simulink model "USV_ASMC"  (R2019b)
settings: Solver=ode1  StartTime=0.0  StopTime=70  FixedStep=0.01  RelTol=1e-3
undefined symbols (not defined in the file): sigbuilder_block
libraries: sharedutil x6, simulink_extras x2, simulink x2, aerolibutil x1
settings Model: Creator=Alex Glz  LastModifiedBy=alex
settings SolverCC: ZeroCrossAlgorithm=Adaptive
settings DataIOCC: ReturnWorkspaceOutputs=off
settings DebuggingCC: IgnoredZcDiagnostic=none  PregeneratedLibrarySubsystemCodeDiagnostic=none  ArithmeticOperatorsInVariantConditions=warning
settings SFSimCC: SimUseLocalCustomCode=off  CustomCodeUndefinedFunction=UseInterfaceOnly
settings RTWCC: RTWUseLocalCustomCode=off

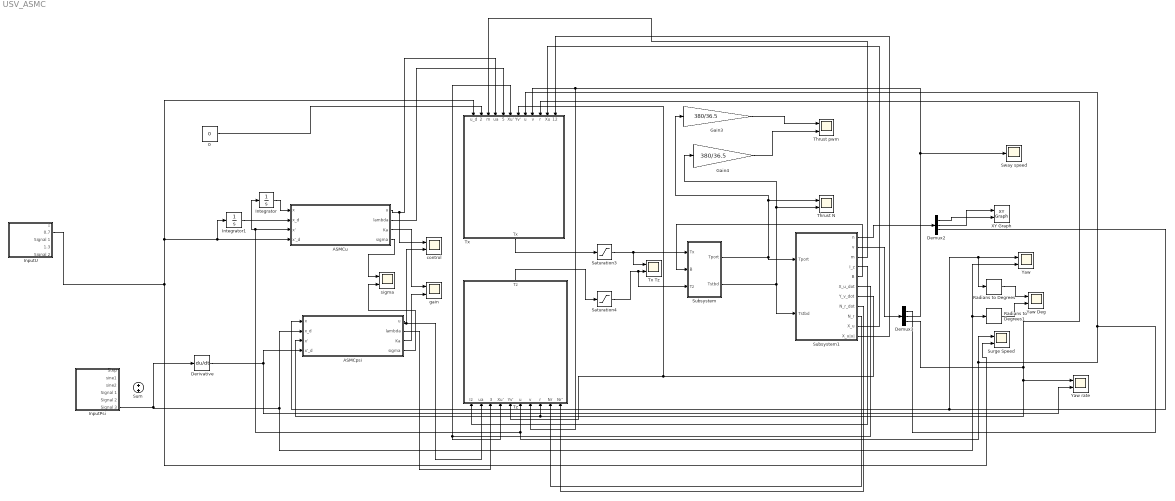
== system USV_ASMC ==
  0 : Constant  Value=0  SampleTime=Inf
  ASMCpsi : Subsystem
  ASMCu : Subsystem
  Demux2 : Demux  Outputs=3
  Demux3 : Demux  Outputs=3
  Derivative : Derivative
  Gain3 : Gain  Gain=380/36.5
  Gain4 : Gain  Gain=380/36.5
  InputPsi : Subsystem  Tag=STV Subsys  LoadFcn=sigbuilder_block('load');  StartFcn=sigbuilder_block('start');  StopFcn=sigbuilder_block('stop');  ClipboardFcn=sigbuilder_block('clipboard');  mask(Sigbuilder block){tuvar=[0:10]}
      mask help: Simulink:masks:SigbuilderBlock_MD
      mask init:
      | if ~strcmp(get_param(bdroot(gcbh),'SimulationStatus'),'stopped') tuvar = sigbuilder_block('maskInit'); end
      settings: CopyFcn=sigbuilder_block('copy');  DeleteFcn=sigbuilder_block('delete');  ModelCloseFcn=sigbuilder_block('modelClose');  PreSaveFcn=sigbuilder_block('preSave');  PauseFcn=sigbuilder_block('pause');  ContinueFcn=sigbuilder_block('continue');  NameChangeFcn=sigbuilder_block('namechange');  OpenFcn=sigbuilder_block('open',[327.411 0 679.074 714.695 ]);  CloseFcn=sigbuilder_block('close');
      mask Display: plot(0, 0, 100, 100,[2, 2, 32, 32, 2], [68, 8, 8, 68, 68],[32, 2], [38, 38], [32, 19, 2],[53, 60, 44], [32, 17, 17, 2],[16, 16, 31, 31]);txt = getActiveGroup(gcbh);text(2, 100, txt,'verticalAlignment', 'top');
  InputU : Subsystem  Tag=STV Subsys  LoadFcn=sigbuilder_block('load');  StartFcn=sigbuilder_block('start');  StopFcn=sigbuilder_block('stop');  ClipboardFcn=sigbuilder_block('clipboard');  mask(Sigbuilder block){tuvar=[0:10]}
      mask help: Simulink:masks:SigbuilderBlock_MD
      mask init:
      | if ~strcmp(get_param(bdroot(gcbh),'SimulationStatus'),'stopped') tuvar = sigbuilder_block('maskInit'); end
      settings: CopyFcn=sigbuilder_block('copy');  DeleteFcn=sigbuilder_block('delete');  ModelCloseFcn=sigbuilder_block('modelClose');  PreSaveFcn=sigbuilder_block('preSave');  PauseFcn=sigbuilder_block('pause');  ContinueFcn=sigbuilder_block('continue');  NameChangeFcn=sigbuilder_block('namechange');  OpenFcn=sigbuilder_block('open',[122.021 0 701.053 737.432 ]);  CloseFcn=sigbuilder_block('close');
      mask Display: plot(0, 0, 100, 100,[2, 2, 32, 32, 2], [68, 8, 8, 68, 68],[32, 2], [38, 38], [32, 19, 2],[53, 60, 44], [32, 17, 17, 2],[16, 16, 31, 31]);txt = getActiveGroup(gcbh);text(2, 100, txt,'verticalAlignment', 'top');
  Integrator : Integrator
  Integrator1 : Integrator
  Radians to Degrees : simulink_extras/Transformations/Radians to Degrees
  Radians to Degrees1 : simulink_extras/Transformations/Radians to Degrees
  Saturation3 : Saturate  UpperLimit=64.97  LowerLimit=-64.97
  Saturation4 : Saturate  UpperLimit=13.31  LowerLimit=-13.31
  Subsystem : Subsystem
  Subsystem1 : Subsystem
  Sum : Sum
  Surge Speed : Scope  NumInputPorts=2
  Sway speed : Scope
  Thrust N : Scope  NumInputPorts=2
  Thrust pwm : Scope  NumInputPorts=2
  Tx : Subsystem
  Tx Tz : Scope  NumInputPorts=2
  Tz : Subsystem
  XY Graph : simulink/Sinks/XY Graph  xmin=-20  xmax=20  ymin=-5  ymax=100  st=-1
  Yaw : Scope  NumInputPorts=2
  Yaw Deg : Scope  NumInputPorts=2
  Yaw rate : Scope  NumInputPorts=2
  control : Scope  NumInputPorts=2
  gain : Scope  NumInputPorts=2
  sigma : Scope  NumInputPorts=2
  wires:
  Subsystem1/1(n) -> Demux2/1
  Subsystem1/2(v) -> Demux3/1
  Gain4/1 -> Thrust pwm/2
  Gain3/1 -> Thrust pwm/1
  Derivative/1 -> ASMCpsi/4(x'_d), Yaw rate/2
  InputU/2(0.7) -> Surge Speed/2, Tx/1(u_d), ASMCu/4(x'_d), Integrator1/1
  Subsystem/2(Tstbd) -> Subsystem1/2(Tstbd), Gain4/1, Thrust N/2
  Subsystem/1(Tport) -> Subsystem1/1(Tport), Thrust N/1, Gain3/1
  Subsystem1/5(B) -> Subsystem/2(B)
  Subsystem1/3(m) -> Tx/3(m)
  ASMCu/1(u) -> control/1, Tx/4(ua)
  ASMCu/2(lambda) -> Tx/5(lambda)
  Subsystem1/6(X_u_dot) -> Tz/4(Xu'), Tx/6(Xu')
  Subsystem1/7(Y_v_dot) -> Tz/5(Yv'), Tx/7(Yv')
  Demux3/1 -> Surge Speed/1, Integrator/1, ASMCu/3(x'), Tz/6(u), Tx/8(u)
  Demux3/2 -> Sway speed/1, Tx/9(v), Tz/7(v)
  Demux3/3 -> Tz/8(r), ASMCpsi/3(x'), Yaw rate/1, Tx/10(r)
  Subsystem1/10(X_u) -> Tx/11(Xu)
  Subsystem1/11(X_u|u|) -> Tx/12(Xu|u|)
  Tx/1(Tx) -> Saturation3/1
  0/1 -> Tx/2(u'_d)
  Subsystem1/4(I_z) -> Tz/1(Iz)
  ASMCpsi/1(u) -> control/2, Tz/2(ua)
  ASMCpsi/2(lambda) -> Tz/3(lambda)
  Subsystem1/9(N_r) -> Tz/9(Nr)
  Subsystem1/8(N_r_dot) -> Tz/10(Nr')
  Tz/1(Tz) -> Saturation4/1
  Demux2/2 -> XY Graph/1
  Demux2/1 -> XY Graph/2
  Radians to Degrees/1 -> Yaw Deg/1
  Radians to Degrees1/1 -> Yaw Deg/2
  Demux2/3 -> Radians to Degrees/1, Yaw/1, ASMCpsi/1(x)
  ASMCu/3(Ka) -> gain/1
  ASMCpsi/3(Ka) -> gain/2
  ASMCu/4(sigma) -> sigma/1
  ASMCpsi/4(sigma) -> sigma/2
  Integrator1/1 -> ASMCu/2(x_d)
  Integrator/1 -> ASMCu/1(x)
  Saturation4/1 -> Subsystem/3(Tz), Tx Tz/2
  Saturation3/1 -> Subsystem/1(Tx), Tx Tz/1
  InputPsi/6(Signal 3) -> ASMCpsi/2(x_d), Yaw/2, Radians to Degrees1/1, Derivative/1

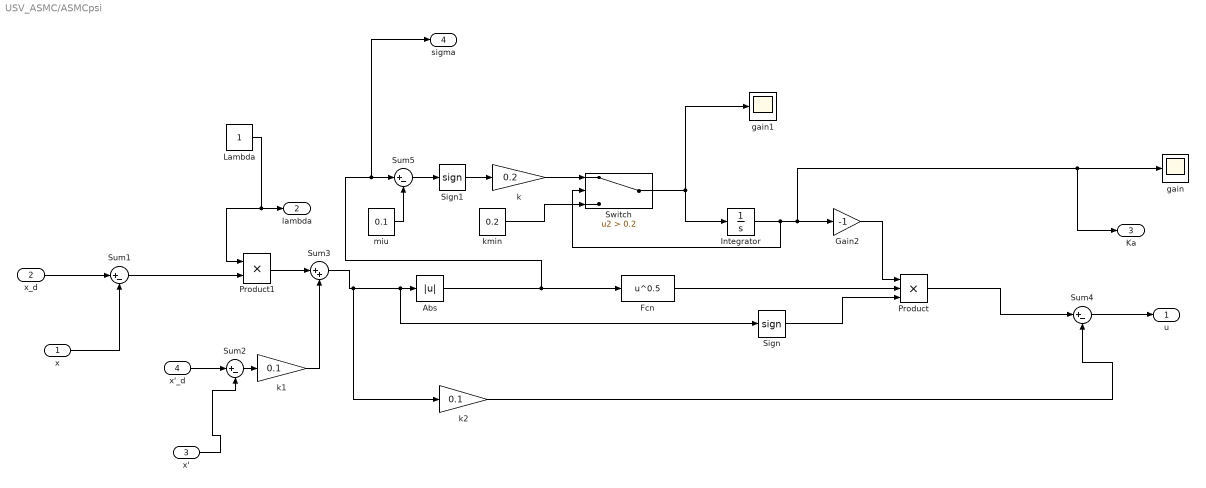
== system USV_ASMC/ASMCpsi ==
  x : Inport
  x_d : Inport  Port=2
  x' : Inport  Port=3
  x'_d : Inport  Port=4
  Abs : Abs
  Fcn : Fcn  Expr=u^0.5
  Gain2 : Gain  Gain=-1
  Integrator : Integrator
  Lambda : Constant
  Product : Product  Inputs=3
  Product1 : Product
  Sign : Signum
  Sign1 : Signum
  Sum{1..2,4..5} (4 alike) : Sum  Inputs=|+-
  Sum3 : Sum  Inputs=|++
  Switch : Switch  Criteria=u2 > Threshold  Threshold=0.2
  gain : Scope
  gain1 : Scope
  k : Gain  Gain=0.2
  k1 : Gain  Gain=0.1
  k2 : Gain  Gain=0.1
  kmin : Constant  Value=0.2
  miu : Constant  Value=0.1
  u : Outport  VectorParamsAs1DForOutWhenUnconnected=off
  lambda : Outport  Port=2  VectorParamsAs1DForOutWhenUnconnected=off
  Ka : Outport  Port=3  VectorParamsAs1DForOutWhenUnconnected=off
  sigma : Outport  Port=4  VectorParamsAs1DForOutWhenUnconnected=off
  wires:
  Product1/1 -> Sum3/1
  x'/1 -> Sum2/2
  x'_d/1 -> Sum2/1
  x_d/1 -> Sum1/1
  x/1 -> Sum1/2
  Sum4/1 -> u/1
  k2/1 -> Sum4/2
  Sum3/1 -> k2/1, Sign/1, Abs/1
  Product/1 -> Sum4/1
  Fcn/1 -> Product/2
  Sign/1 -> Product/3
  Gain2/1 -> Product/1
  Integrator/1 -> Switch/2, Ka/1, gain/1, Gain2/1
  miu/1 -> Sum5/2
  Sum5/1 -> Sign1/1
  Sign1/1 -> k/1
  k/1 -> Switch/1
  Switch/1 -> gain1/1, Integrator/1
  kmin/1 -> Switch/3
  Lambda/1 -> Product1/1, lambda/1
  Sum1/1 -> Product1/2
  Sum2/1 -> k1/1
  Abs/1 -> sigma/1, Sum5/1, Fcn/1
  k1/1 -> Sum3/2

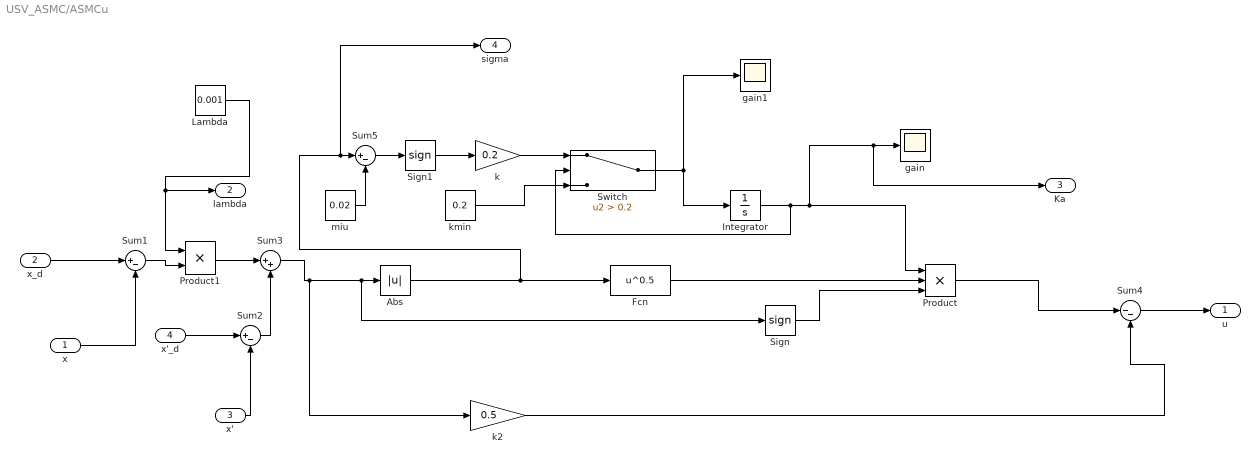
== system USV_ASMC/ASMCu ==
  x : Inport
  x_d : Inport  Port=2
  x' : Inport  Port=3
  x'_d : Inport  Port=4
  Abs : Abs
  Fcn : Fcn  Expr=u^0.5
  Integrator : Integrator
  Lambda : Constant  Value=0.001
  Product : Product  Inputs=3
  Product1 : Product
  Sign : Signum
  Sign1 : Signum
  Sum1 : Sum  Inputs=|+-
  Sum2 : Sum  Inputs=|+-
  Sum3 : Sum  Inputs=|++
  Sum4 : Sum  Inputs=|--
  Sum5 : Sum  Inputs=|+-
  Switch : Switch  Criteria=u2 > Threshold  Threshold=0.2
  gain : Scope
  gain1 : Scope
  k : Gain  Gain=0.2
  k2 : Gain  Gain=0.5
  kmin : Constant  Value=0.2
  miu : Constant  Value=0.02
  u : Outport  VectorParamsAs1DForOutWhenUnconnected=off
  lambda : Outport  Port=2  VectorParamsAs1DForOutWhenUnconnected=off
  Ka : Outport  Port=3  VectorParamsAs1DForOutWhenUnconnected=off
  sigma : Outport  Port=4  VectorParamsAs1DForOutWhenUnconnected=off
  wires:
  Product1/1 -> Sum3/1
  x'/1 -> Sum2/2
  x'_d/1 -> Sum2/1
  Sum2/1 -> Sum3/2
  x_d/1 -> Sum1/1
  x/1 -> Sum1/2
  Sum1/1 -> Product1/2
  Sum4/1 -> u/1
  k2/1 -> Sum4/2
  Sum3/1 -> k2/1, Sign/1, Abs/1
  Product/1 -> Sum4/1
  Fcn/1 -> Product/2
  Sign/1 -> Product/3
  Integrator/1 -> Switch/2, Product/1, Ka/1, gain/1
  miu/1 -> Sum5/2
  Sum5/1 -> Sign1/1
  Sign1/1 -> k/1
  k/1 -> Switch/1
  Switch/1 -> gain1/1, Integrator/1
  kmin/1 -> Switch/3
  Lambda/1 -> lambda/1, Product1/1
  Abs/1 -> sigma/1, Sum5/1, Fcn/1

== system USV_ASMC/InputPsi ==
  Demux : Demux  Tag=STV Demux  Outputs=6
  FromWs : FromWorkspace  Tag=STV FromWs  VariableName=tuvar  SampleTime=0
      SigBuilderData=|
      | common.afterFinalStr = 'Extrapolate'
      | common.sampleTime = 0
      | dataSet.timeRange = [0 90]
      | dataSet.name = 'Group 1'
      | sbobj.Groups.Name = 'Group 1'
      | sbobj.Groups.Signals(1).Name = 'Step'
      | sbobj.Groups.Signals(1).XData = [0 90]
      | sbobj.Groups.Signals(1).YData = [0.4 0.4]
      | sbobj.Groups.Signals(2).Name = 'sine1'
      | sbobj.Groups.Signals(2).XData = [0 2.94117647059 5.88235294118 8.82352941176 11.7647058824 14.7058823529 17.6470588235 20.5882352941 23.5294117647 26.4705882353 29.4117647059 32.3529411765 35.2941176471 38.2352941176 41.1764705882 44.1176470588 47.0588235294 50 90]
      | sbobj.Groups.Signals(2).YData = [0 0.144496666475 0.269478257459 0.358065316542 0.398293670518 0.384730257269 0.319206890912 0.210572865151 0.0734998071266 -0.0734998071266 -0.210572865151 -0.319206890912 -0.384730257269 -0.398293670518 -0.358065316542 -0.269478257459 -0.144496666475 0 0]
      | sbobj.Groups.Signals(3).Name = 'sine2'
      | sbobj.Groups.Signals(3).XData = [0 2.94117647059 5.88235294118 8.82352941176 11.7647058824 14.7058823529 17.6470588235 20.5882352941 23.5294117647 26.4705882353 29.4117647059 32.3529411765 35.2941176471 38.2352941176 41.1764705882 44.1176470588 45 50 90]
      | sbobj.Groups.Signals(3).YData = [0 0.0722483332374 0.134739128729 0.179032658271 0.199146835259 0.192365128635 0.159603445456 0.105286432575 0.0367499035633 -0.0367499035633 -0.105286432575 -0.159603445456 -0.192365128635 -0.199146835259 -0.179032658271 -0.134739128729 -0.117557050458 0 0]
      | sbobj.Groups.Signals(4).Name = 'Signal 1'
      | sbobj.Groups.Signals(4).XData = [0 30 30 50 60 60 90]
      | sbobj.Groups.Signals(4).YData = [3 3 2 2 2 1 1]
      | sbobj.Groups.Signals(5).Name = 'Signal 2'
      | sbobj.Groups.Signals(5).XData = [0 0.01 0.02 0.03 0.04 0.05 0.06 0.07 0.08 0.09 0.1 0.11 ... (9001 elements, 1x9001)]
      | sbobj.Groups.Signals(5).YData = [-0.0197341459996 0.0101006698948 0.00109159685548 0.00682613120581 -0.00894223767885 0.0161354484461 -0.00589998785907 0.00664245185836 -0.0112621395209 -0.00996625777906 -0.00906837882606 -0.00281492525369 ... (9001 elements, 1x9001)]
      | sbobj.Groups.Signals(6).Name = 'Signal 3'
      | sbobj.Groups.Signals(6).XData = [0 0.0625625625626 0.125125125125 0.187687687688 0.25025025025 0.312812812813 0.375375375375 0.437937937938 0.500500500501 0.563063063063 0.625625625626 0.688188188188 ... (1440 elements, 1x1440)]
      | sbobj.Groups.Signals(6).YData = [0 0.0157235832902 0.0314465445969 0.0471682619612 0.0628881134734 0.0786054772978 0.0943197316968 0.110030255056 0.125736425908 0.141437622959 0.157133225111 0.172822611487 ... (1440 elements, 1x1440)]
      | sbobj.Groups.TimeRange = [0 90]
  Step : Outport  Tag=STV Outport  VectorParamsAs1DForOutWhenUnconnected=off
  sine1 : Outport  Tag=STV Outport  Port=2  VectorParamsAs1DForOutWhenUnconnected=off
  sine2 : Outport  Tag=STV Outport  Port=3  VectorParamsAs1DForOutWhenUnconnected=off
  Signal 1 : Outport  Tag=STV Outport  Port=4  VectorParamsAs1DForOutWhenUnconnected=off
  Signal 2 : Outport  Tag=STV Outport  Port=5  VectorParamsAs1DForOutWhenUnconnected=off
  Signal 3 : Outport  Tag=STV Outport  Port=6
  wires:
  FromWs/1 -> Demux/1
  Demux/1 -> Step/1
  Demux/2 -> sine1/1
  Demux/3 -> sine2/1
  Demux/4 -> Signal 1/1
  Demux/5 -> Signal 2/1
  Demux/6 -> Signal 3/1

== system USV_ASMC/InputU ==
  Demux : Demux  Tag=STV Demux  Outputs=5
  FromWs : FromWorkspace  Tag=STV FromWs  VariableName=tuvar  SampleTime=0
      SigBuilderData=|
      | common.afterFinalStr = 'Extrapolate'
      | common.sampleTime = 0
      | dataSet.timeRange = [0 45]
      | dataSet.name = 'Group 1'
      | sbobj.Groups.Name = 'Group 1'
      | sbobj.Groups.Signals(1).Name = '1'
      | sbobj.Groups.Signals(1).XData = [0 45]
      | sbobj.Groups.Signals(1).YData = [1 1]
      | sbobj.Groups.Signals(2).Name = '0.7'
      | sbobj.Groups.Signals(2).XData = [0 45]
      | sbobj.Groups.Signals(2).YData = [0.7 0.7]
      | sbobj.Groups.Signals(3).Name = 'Signal 1'
      | sbobj.Groups.Signals(3).XData = [0 2.94117647059 5.88235294118 8.82352941176 11.7647058824 14.7058823529 17.6470588235 20.5882352941 23.5294117647 26.4705882353 29.4117647059 32.3529411765 35.2941176471 38.2352941176 41.1764705882 44.1176470588 45]
      | sbobj.Groups.Signals(3).YData = [0 0.680620833094 0.836847821823 0.947581645678 0.997867088148 0.980912821586 0.89900861364 0.763216081439 0.591874758908 0.408125241092 0.236783918561 0.10099138636 0.0190871784136 0 0 0 0]
      | sbobj.Groups.Signals(4).Name = '1.3'
      | sbobj.Groups.Signals(4).XData = [0 45]
      | sbobj.Groups.Signals(4).YData = [1.3 1.3]
      | sbobj.Groups.Signals(5).Name = 'Signal 2'
      | sbobj.Groups.Signals(5).XData = [0 2.94117647059 5.88235294118 8.82352941176 11.7647058824 14.7058823529 17.6470588235 20.5882352941 23.5294117647 26.4705882353 45]
      | sbobj.Groups.Signals(5).YData = [0 0.680620833094 0.836847821823 0.947581645678 0.997867088148 0.980912821586 0.89900861364 0.763216081439 0.591874758908 0.5 0.5]
      | sbobj.Groups.TimeRange = [0 45]
  1 : Outport  Tag=STV Outport  VectorParamsAs1DForOutWhenUnconnected=off
  0.7 : Outport  Tag=STV Outport  Port=2  VectorParamsAs1DForOutWhenUnconnected=off
  Signal 1 : Outport  Tag=STV Outport  Port=3  VectorParamsAs1DForOutWhenUnconnected=off
  1.3 : Outport  Tag=STV Outport  Port=4  VectorParamsAs1DForOutWhenUnconnected=off
  Signal 2 : Outport  Tag=STV Outport  Port=5  VectorParamsAs1DForOutWhenUnconnected=off
  wires:
  FromWs/1 -> Demux/1
  Demux/1 -> 1/1
  Demux/2 -> 0.7/1
  Demux/3 -> Signal 1/1
  Demux/4 -> 1.3/1
  Demux/5 -> Signal 2/1

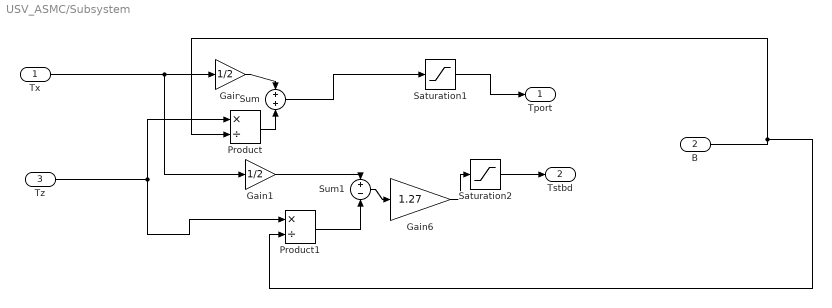
== system USV_ASMC/Subsystem ==
  Tx : Inport
  B : Inport  Port=2
  Tz : Inport  Port=3
  Gain : Gain  Gain=1/2
  Gain1 : Gain  Gain=1/2
  Gain6 : Gain  Gain=1.27
  Product : Product  Inputs=*/
  Product1 : Product  Inputs=*/
  Saturation1 : Saturate  UpperLimit=36.5  LowerLimit=-30
  Saturation2 : Saturate  UpperLimit=36.5  LowerLimit=-30
  Sum : Sum
  Sum1 : Sum  Inputs=+-
  Tport : Outport  VectorParamsAs1DForOutWhenUnconnected=off
  Tstbd : Outport  Port=2  VectorParamsAs1DForOutWhenUnconnected=off
  wires:
  Gain6/1 -> Saturation2/1
  Gain/1 -> Sum/1
  Sum/1 -> Saturation1/1
  B/1 -> Product/2, Product1/2
  Tz/1 -> Product1/1, Product/1
  Saturation1/1 -> Tport/1
  Product/1 -> Sum/2
  Tx/1 -> Gain1/1, Gain/1
  Product1/1 -> Sum1/2
  Saturation2/1 -> Tstbd/1
  Gain1/1 -> Sum1/1
  Sum1/1 -> Gain6/1

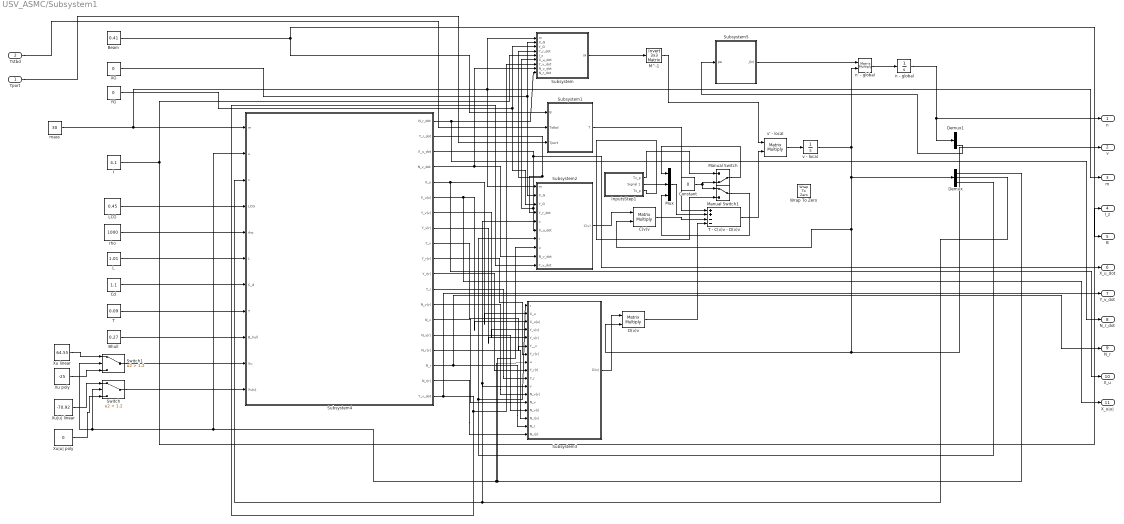
== system USV_ASMC/Subsystem1 ==
  Tport : Inport
  Tstbd : Inport  Port=2
  Beam : Constant  Value=0.41
  "Bhull " : Constant  Value=0.27
  C(v)v : Product  Multiplication=Matrix(*)
  Cd : Constant  Value=1.1
  Constant : Constant  Value=0
  D(v)v : Product  Multiplication=Matrix(*)
  Demux : Demux  Outputs=3
  Demux1 : Demux  Outputs=3
  "I " : Constant  Value=4.1
  InputsStep1 : Subsystem  Tag=STV Subsys  LoadFcn=sigbuilder_block('load');  StartFcn=sigbuilder_block('start');  StopFcn=sigbuilder_block('stop');  ClipboardFcn=sigbuilder_block('clipboard');  mask(Sigbuilder block){tuvar=[0:10]}
      mask help: Simulink:masks:SigbuilderBlock_MD
      mask init:
      | if ~strcmp(get_param(bdroot(gcbh),'SimulationStatus'),'stopped') tuvar = sigbuilder_block('maskInit'); end
      settings: CopyFcn=sigbuilder_block('copy');  DeleteFcn=sigbuilder_block('delete');  ModelCloseFcn=sigbuilder_block('modelClose');  PreSaveFcn=sigbuilder_block('preSave');  PauseFcn=sigbuilder_block('pause');  ContinueFcn=sigbuilder_block('continue');  NameChangeFcn=sigbuilder_block('namechange');  OpenFcn=sigbuilder_block('open',[233.25 0 805.5 688.168 ]);  CloseFcn=sigbuilder_block('close');
      mask Display: plot(0, 0, 100, 100,[2, 2, 32, 32, 2], [68, 8, 8, 68, 68],[32, 2], [38, 38], [32, 19, 2],[53, 60, 44], [32, 17, 17, 2],[16, 16, 31, 31]);txt = getActiveGroup(gcbh);text(2, 100, txt,'verticalAlignment', 'top');
  L : Constant  Value=1.01
  LCG : Constant  Value=0.45
  M^-1 : aerolibutil/Invert  3x3 Matrix
  Manual Switch : ManualSwitch  CurrentSetting=0
  Manual Switch1 : ManualSwitch
  Mux : Mux  Inputs=3
  Subsystem : Subsystem
  Subsystem1 : Subsystem
  Subsystem2 : Subsystem
  Subsystem3 : Subsystem
  Subsystem4 : Subsystem
  Subsystem5 : Subsystem
  Switch : Switch  Criteria=u2 > Threshold  Threshold=1.2
  Switch1 : Switch  Criteria=u2 > Threshold  Threshold=1.2
  T : Constant  Value=0.09
  T - C(v)v - D(v)v : Sum  Inputs=++--
  Wrap To Zero : simulink/Discontinuities/Wrap To Zero  Threshold=255
      settings: SourceProductName=Simulink  SourceProductBaseCode=SL
  XG : Constant  Value=0
  Xu linear : Constant  Value=64.55
  Xu poly : Constant  Value=-25
  Xu|u| linear : Constant  Value=-70.92
  Xu|u| poly : Constant  Value=0
  YG : Constant  Value=0
  mass : Constant  Value=30
  n - global : Integrator  InitialCondition=[0 0 0]
  n' - global : Product  Multiplication=Matrix(*)
  rho : Constant  Value=1000
  v - local : Integrator
  v' - local : Product  Multiplication=Matrix(*)
  n : Outport  VectorParamsAs1DForOutWhenUnconnected=off
  v : Outport  Port=2  VectorParamsAs1DForOutWhenUnconnected=off
  m : Outport  Port=3  VectorParamsAs1DForOutWhenUnconnected=off
  I_z : Outport  Port=4  VectorParamsAs1DForOutWhenUnconnected=off
  B : Outport  Port=5  VectorParamsAs1DForOutWhenUnconnected=off
  X_u_dot : Outport  Port=6  VectorParamsAs1DForOutWhenUnconnected=off
  Y_v_dot : Outport  Port=7  VectorParamsAs1DForOutWhenUnconnected=off
  N_r_dot : Outport  Port=8  VectorParamsAs1DForOutWhenUnconnected=off
  N_r : Outport  Port=9  VectorParamsAs1DForOutWhenUnconnected=off
  X_u : Outport  Port=10  VectorParamsAs1DForOutWhenUnconnected=off
  X_u|u| : Outport  Port=11  VectorParamsAs1DForOutWhenUnconnected=off
  wires:
  Subsystem4/3(X_u_dot) -> X_u_dot/1, Subsystem2/6(X_u_dot), Subsystem/6(X_u_dot)
  mass/1 -> m/1, Subsystem2/1(m), Subsystem/1(m), Subsystem4/1(m)
  M^-1/1 -> v' - local/1
  Demux/3 -> Subsystem3/1(r), Subsystem2/7(r)
  Subsystem4/17(N_r) -> N_r/1, Subsystem3/16(N_r)
  L/1 -> Subsystem4/6(L)
  Subsystem4/4(N_v_dot) -> Subsystem2/9(N_v_dot), Subsystem/8(N_v_dot)
  v - local/1 -> v/1, D(v)v/2, C(v)v/2, Demux/1, n' - global/2
  "Bhull "/1 -> Subsystem4/9(B_hull)
  T/1 -> Subsystem4/8(T)
  Demux/1 -> Switch/2, Switch1/2, Subsystem4/2(u), Subsystem3/8(u), Subsystem2/8(u)
  YG/1 -> Subsystem2/3(Y_G), Subsystem/3(Y_G)
  Xu linear/1 -> Switch1/1
  Demux/2 -> Subsystem4/3(v), Subsystem2/5(v), Subsystem3/11(v)
  Subsystem4/2(Y_r_dot) -> Subsystem/4(Y_r_dot), Subsystem2/4(Y_r_dot)
  Subsystem3/1(D(v)) -> D(v)v/1
  XG/1 -> Subsystem2/2(X_G), Subsystem/2(X_G)
  n' - global/1 -> n - global/1
  Subsystem4/19(Y_v_dot) -> Y_v_dot/1, Subsystem2/10(Y_v_dot), Subsystem/7(Y_v_dot)
  Cd/1 -> Subsystem4/7(C_d)
  Tstbd/1 -> Subsystem1/2(Tstbd)
  Subsystem/1(M) -> M^-1/1
  Subsystem4/15(N_v|r|) -> Subsystem3/14(N_v|r|)
  n - global/1 -> n/1, Demux1/1
  Beam/1 -> B/1, Subsystem1/1(B)
  Tport/1 -> Subsystem1/3(Tport)
  Subsystem1/1(T) -> T - C(v)v - D(v)v/1
  LCG/1 -> Subsystem4/4(LCG)
  Subsystem4/12(Y_r) -> Subsystem3/10(Y_r)
  C(v)v/1 -> T - C(v)v - D(v)v/3
  rho/1 -> Subsystem4/5(rho)
  Subsystem4/1(N_r_dot) -> N_r_dot/1, Subsystem/9(N_r_dot)
  D(v)v/1 -> T - C(v)v - D(v)v/4
  T - C(v)v - D(v)v/1 -> v' - local/2
  Subsystem4/8(Y_v|r|) -> Subsystem3/5(Y_v|r|)
  Subsystem4/18(N_r|r|) -> Subsystem3/17(N_r|r|)
  Subsystem4/11(Y_r|r|) -> Subsystem3/9(Y_r|r|)
  Xu|u| linear/1 -> Switch/1
  Switch1/1 -> Subsystem4/10(Xu)
  Subsystem4/13(N_v|v|) -> Subsystem3/12(N_v|v|)
  Switch/1 -> Subsystem4/11(Xu|u|)
  Subsystem4/7(Y_v|v|) -> Subsystem3/4(Y_v|v|)
  Subsystem4/6(X_u|u|) -> X_u|u|/1, Subsystem3/3(X_u|u|)
  Subsystem4/10(Y_r|v|) -> Subsystem3/7(Y_r|v|)
  Subsystem4/5(X_u) -> X_u/1, Subsystem3/2(X_u)
  "I "/1 -> I_z/1, Subsystem/5(I_z)
  Subsystem2/1(C(v)) -> C(v)v/1
  Subsystem4/9(Y_v) -> Subsystem3/6(Y__v)
  v' - local/1 -> v - local/1
  Subsystem4/16(N_r|v|) -> Subsystem3/15(N_r|v|)
  Subsystem5/1(J(n)) -> n' - global/1
  Subsystem4/14(N_v) -> Subsystem3/13(N_v)
  Xu poly/1 -> Switch1/3
  Xu|u| poly/1 -> Switch/3
  Demux1/3 -> Subsystem5/1(psi)
  InputsStep1/2(Signal 1) -> Mux/2
  Manual Switch/1 -> Mux/1
  Manual Switch1/1 -> Mux/3
  Mux/1 -> T - C(v)v - D(v)v/2
  InputsStep1/3(Tz_p) -> Manual Switch1/2
  InputsStep1/1(Tx_p) -> Manual Switch/1
  Constant/1 -> Manual Switch/2, Manual Switch1/1

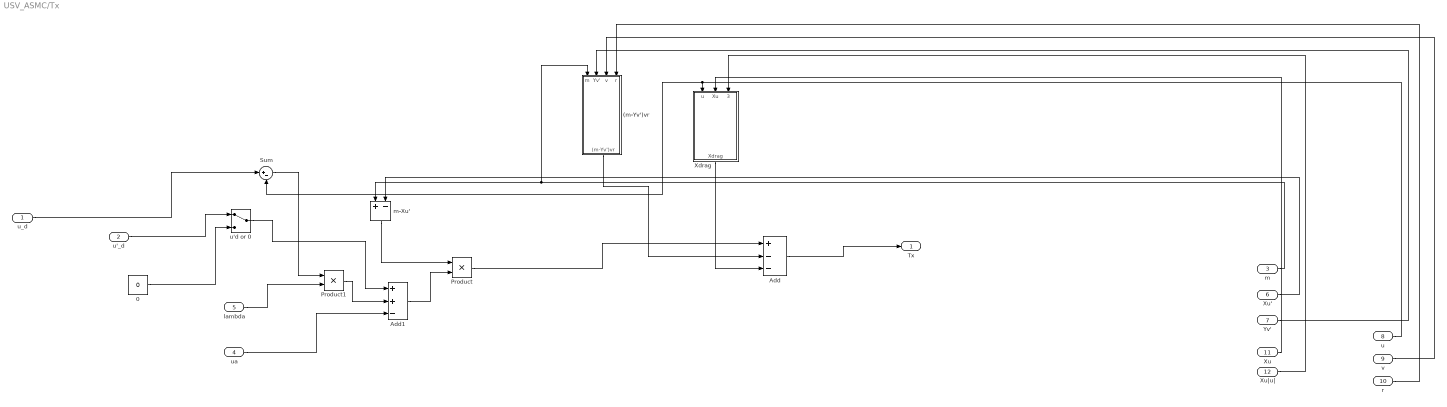
== system USV_ASMC/Tx ==
  u_d : Inport
  u'_d : Inport  Port=2
  m : Inport  Port=3
  ua : Inport  Port=4
  lambda : Inport  Port=5
  Xu' : Inport  Port=6
  Yv' : Inport  Port=7
  u : Inport  Port=8
  v : Inport  Port=9
  r : Inport  Port=10
  Xu : Inport  Port=11
  Xu|u| : Inport  Port=12
  (m-Yv')vr : Subsystem
  0 : Constant  Value=0  SampleTime=Inf
  Add : Sum  Inputs=+--
  Add1 : Sum  Inputs=++-
  Product : Product
  Product1 : Product
  Sum : Sum  Inputs=|+-
  Xdrag : Subsystem
  m-Xu' : Sum  Inputs=+-
  u'd or 0 : ManualSwitch
  Tx : Outport  VectorParamsAs1DForOutWhenUnconnected=off
  wires:
  Xu/1 -> Xdrag/2(Xu)
  ua/1 -> Add1/3
  Yv'/1 -> (m-Yv')vr/2(Yv')
  Sum/1 -> Product1/1
  Product1/1 -> Add1/2
  r/1 -> (m-Yv')vr/4(r)
  Xu|u|/1 -> Xdrag/3(Xu|u|)
  (m-Yv')vr/1((m-Yv')vr) -> Add/2
  Add/1 -> Tx/1
  m-Xu'/1 -> Product/1
  u'_d/1 -> u'd or 0/1
  v/1 -> (m-Yv')vr/3(v)
  m/1 -> m-Xu'/1, (m-Yv')vr/1(m)
  u_d/1 -> Sum/1
  lambda/1 -> Product1/2
  Xdrag/1(Xdrag) -> Add/3
  Product/1 -> Add/1
  Add1/1 -> Product/2
  u/1 -> Sum/2, Xdrag/1(u)
  Xu'/1 -> m-Xu'/2
  u'd or 0/1 -> Add1/1
  0/1 -> u'd or 0/2

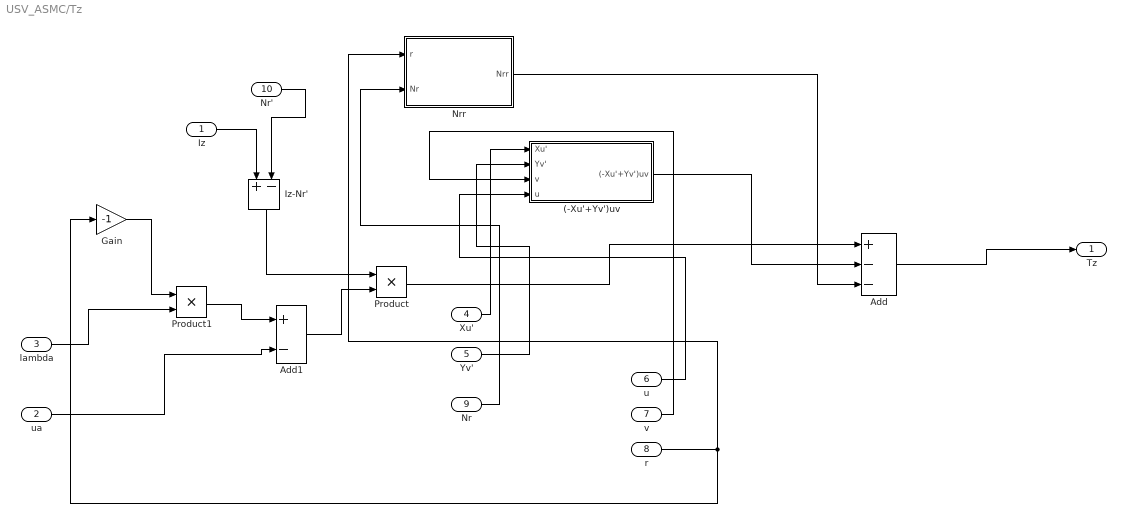
== system USV_ASMC/Tz ==
  Iz : Inport
  ua : Inport  Port=2
  lambda : Inport  Port=3
  Xu' : Inport  Port=4
  Yv' : Inport  Port=5
  u : Inport  Port=6
  v : Inport  Port=7
  r : Inport  Port=8
  Nr : Inport  Port=9
  Nr' : Inport  Port=10
  (-Xu'+Yv')uv : Subsystem
  Add : Sum  Inputs=+--
  Add1 : Sum  Inputs=+-
  Gain : Gain  Gain=-1
  Iz-Nr' : Sum  Inputs=+-
  Nrr : Subsystem
  Product : Product
  Product1 : Product
  Tz : Outport  VectorParamsAs1DForOutWhenUnconnected=off
  wires:
  Nr/1 -> Nrr/2(Nr)
  ua/1 -> Add1/2
  Yv'/1 -> (-Xu'+Yv')uv/2(Yv')
  Product1/1 -> Add1/1
  r/1 -> Gain/1, Nrr/1(r)
  (-Xu'+Yv')uv/1((-Xu'+Yv')uv) -> Add/2
  Add/1 -> Tz/1
  Iz-Nr'/1 -> Product/1
  v/1 -> (-Xu'+Yv')uv/3(v)
  Iz/1 -> Iz-Nr'/1
  lambda/1 -> Product1/2
  Nrr/1(Nrr) -> Add/3
  Product/1 -> Add/1
  Add1/1 -> Product/2
  u/1 -> (-Xu'+Yv')uv/4(u)
  Xu'/1 -> (-Xu'+Yv')uv/1(Xu')
  Nr'/1 -> Iz-Nr'/2
  Gain/1 -> Product1/1

== system USV_ASMC/Subsystem1/InputsStep1 ==
  Demux : Demux  Tag=STV Demux  Outputs=3
  FromWs : FromWorkspace  Tag=STV FromWs  VariableName=tuvar  SampleTime=0
      SigBuilderData=|
      | common.afterFinalStr = 'Extrapolate'
      | common.sampleTime = 0
      | dataSet.timeRange = [0 45]
      | dataSet.name = 'Group 1'
      | sbobj.Groups.Name = 'Group 1'
      | sbobj.Groups.Signals(1).Name = 'Tx_p'
      | sbobj.Groups.Signals(1).XData = [0 15 15 45]
      | sbobj.Groups.Signals(1).YData = [0 0 -5 -5]
      | sbobj.Groups.Signals(2).Name = 'Signal 1'
      | sbobj.Groups.Signals(2).XData = [0 45]
      | sbobj.Groups.Signals(2).YData = [0 0]
      | sbobj.Groups.Signals(3).Name = 'Tz_p'
      | sbobj.Groups.Signals(3).XData = [0 15 15 40 40 45]
      | sbobj.Groups.Signals(3).YData = [0 0 1 1 0 0]
      | sbobj.Groups.TimeRange = [0 45]
  Tx_p : Outport  Tag=STV Outport  VectorParamsAs1DForOutWhenUnconnected=off
  Signal 1 : Outport  Tag=STV Outport  Port=2  VectorParamsAs1DForOutWhenUnconnected=off
  Tz_p : Outport  Tag=STV Outport  Port=3  VectorParamsAs1DForOutWhenUnconnected=off
  wires:
  FromWs/1 -> Demux/1
  Demux/1 -> Tx_p/1
  Demux/2 -> Signal 1/1
  Demux/3 -> Tz_p/1

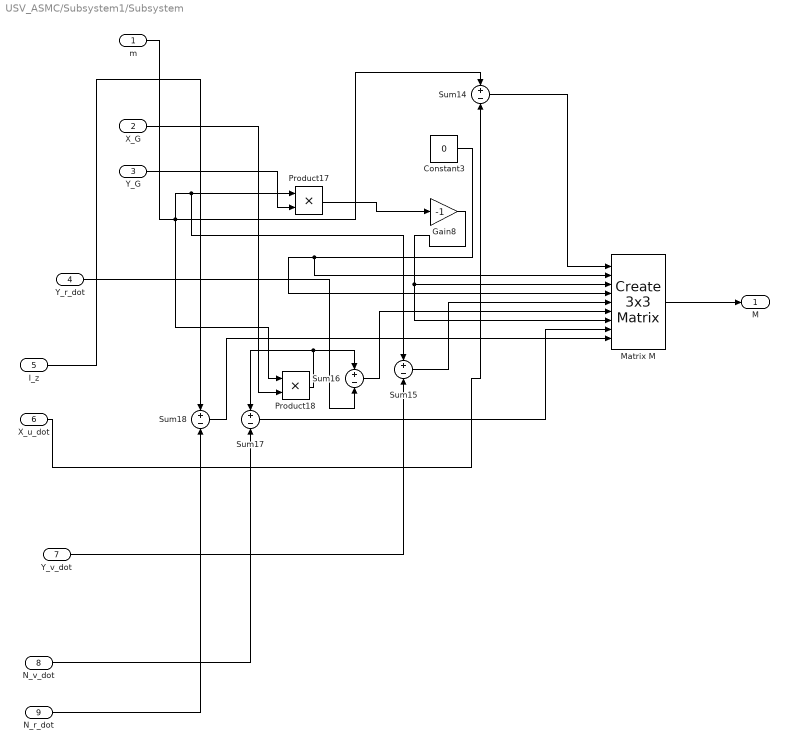
== system USV_ASMC/Subsystem1/Subsystem ==
  m : Inport
  X_G : Inport  Port=2
  Y_G : Inport  Port=3
  Y_r_dot : Inport  Port=4
  I_z : Inport  Port=5
  X_u_dot : Inport  Port=6
  Y_v_dot : Inport  Port=7
  N_v_dot : Inport  Port=8
  N_r_dot : Inport  Port=9
  Constant3 : Constant  Value=0
  Gain8 : Gain  Gain=-1
  Matrix M : sharedutil/Create 3x3 Matrix  aMode=aMode
  Product17 : Product
  Product18 : Product
  Sum{14..18} (5 alike) : Sum  Inputs=+-
  M : Outport  VectorParamsAs1DForOutWhenUnconnected=off
  wires:
  Gain8/1 -> Matrix M/7, Matrix M/3
  Product17/1 -> Gain8/1
  Product18/1 -> Sum17/1, Sum16/1
  Sum18/1 -> Matrix M/9
  Constant3/1 -> Matrix M/4, Matrix M/2
  I_z/1 -> Sum18/1
  Sum15/1 -> Matrix M/5
  Y_v_dot/1 -> Sum15/2
  m/1 -> Sum15/1, Product17/1, Product18/1, Sum14/1
  N_v_dot/1 -> Sum17/2
  Sum14/1 -> Matrix M/1
  Sum16/1 -> Matrix M/6
  Matrix M/1 -> M/1
  Sum17/1 -> Matrix M/8
  X_G/1 -> Product18/2
  Y_G/1 -> Product17/2
  Y_r_dot/1 -> Sum16/2
  X_u_dot/1 -> Sum14/2
  N_r_dot/1 -> Sum18/2

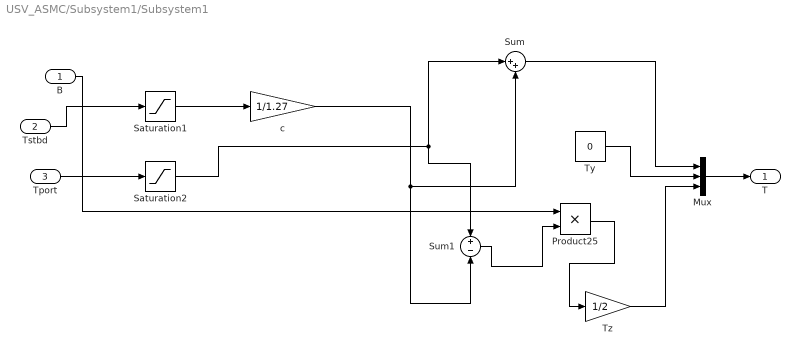
== system USV_ASMC/Subsystem1/Subsystem1 ==
  B : Inport
  Tstbd : Inport  Port=2
  Tport : Inport  Port=3
  Mux : Mux  Inputs=3
  Product25 : Product
  Saturation1 : Saturate  UpperLimit=36.5  LowerLimit=-30
  Saturation2 : Saturate  UpperLimit=36.5  LowerLimit=-30
  Sum : Sum  Inputs=|++
  Sum1 : Sum  Inputs=+-
  Ty : Constant  Value=0
  Tz : Gain  Gain=1/2
  c : Gain  Gain=1/1.27
  T : Outport  VectorParamsAs1DForOutWhenUnconnected=off
  wires:
  Sum/1 -> Mux/1
  Tstbd/1 -> Saturation1/1
  Ty/1 -> Mux/2
  Sum1/1 -> Product25/2
  B/1 -> Product25/1
  Mux/1 -> T/1
  Tz/1 -> Mux/3
  Product25/1 -> Tz/1
  Tport/1 -> Saturation2/1
  c/1 -> Sum1/2, Sum/2
  Saturation1/1 -> c/1
  Saturation2/1 -> Sum1/1, Sum/1

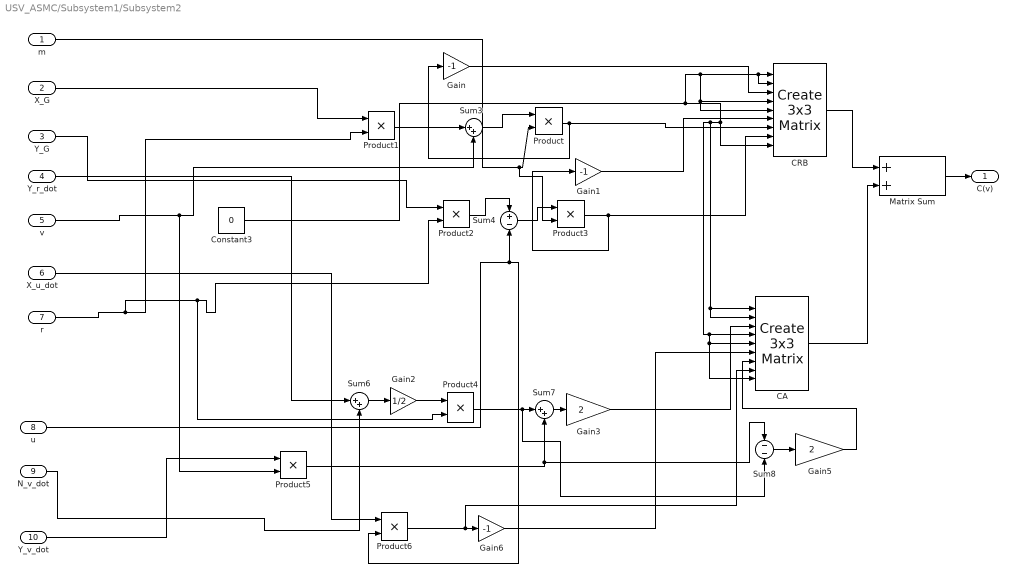
== system USV_ASMC/Subsystem1/Subsystem2 ==
  m : Inport
  X_G : Inport  Port=2
  Y_G : Inport  Port=3
  Y_r_dot : Inport  Port=4
  v : Inport  Port=5
  X_u_dot : Inport  Port=6
  r : Inport  Port=7
  u : Inport  Port=8
  N_v_dot : Inport  Port=9
  Y_v_dot : Inport  Port=10
  " CRB" : sharedutil/Create 3x3 Matrix  aMode=aMode
  CA : sharedutil/Create 3x3 Matrix  aMode=aMode
  Constant3 : Constant  Value=0
  Gain : Gain  Gain=-1
  Gain1 : Gain  Gain=-1
  Gain2 : Gain  Gain=1/2
  Gain3 : Gain  Gain=2
  Gain5 : Gain  Gain=2
  Gain6 : Gain  Gain=-1
  Matrix Sum : Sum
  Product{,1..6} (7 alike) : Product
  Sum3 : Sum  Inputs=|++
  Sum4 : Sum  Inputs=+-
  Sum6 : Sum  Inputs=|++
  Sum7 : Sum  Inputs=|++
  Sum8 : Sum  Inputs=--
  C(v) : Outport  VectorParamsAs1DForOutWhenUnconnected=off
  wires:
  Constant3/1 -> CA/9, CA/5, CA/4, CA/2, CA/1, " CRB"/9, " CRB"/2, " CRB"/1, " CRB"/5, " CRB"/4
  m/1 -> Product3/2, Product/2
  Product/1 -> Gain/1, " CRB"/7
  Sum7/1 -> Gain3/1
  X_G/1 -> Product1/1
  u/1 -> Product6/2, Sum4/2
  " CRB"/1 -> Matrix Sum/1
  Gain5/1 -> CA/7
  Product3/1 -> Gain1/1, " CRB"/8
  Product4/1 -> Sum8/2, Sum7/1
  v/1 -> Sum3/2, Product5/2
  Product6/1 -> CA/8, Gain6/1
  Gain6/1 -> CA/6
  Gain3/1 -> CA/3
  Matrix Sum/1 -> C(v)/1
  Y_G/1 -> Product2/1
  Product1/1 -> Sum3/1
  Gain1/1 -> " CRB"/6
  Product5/1 -> Sum8/1, Sum7/2
  Sum6/1 -> Gain2/1
  Product2/1 -> Sum4/1
  Sum4/1 -> Product3/1
  Sum8/1 -> Gain5/1
  Sum3/1 -> Product/1
  X_u_dot/1 -> Product6/1
  N_v_dot/1 -> Sum6/2
  Gain/1 -> " CRB"/3
  CA/1 -> Matrix Sum/2
  Gain2/1 -> Product4/1
  r/1 -> Product2/2, Product4/2, Product1/2
  Y_v_dot/1 -> Product5/1
  Y_r_dot/1 -> Sum6/1

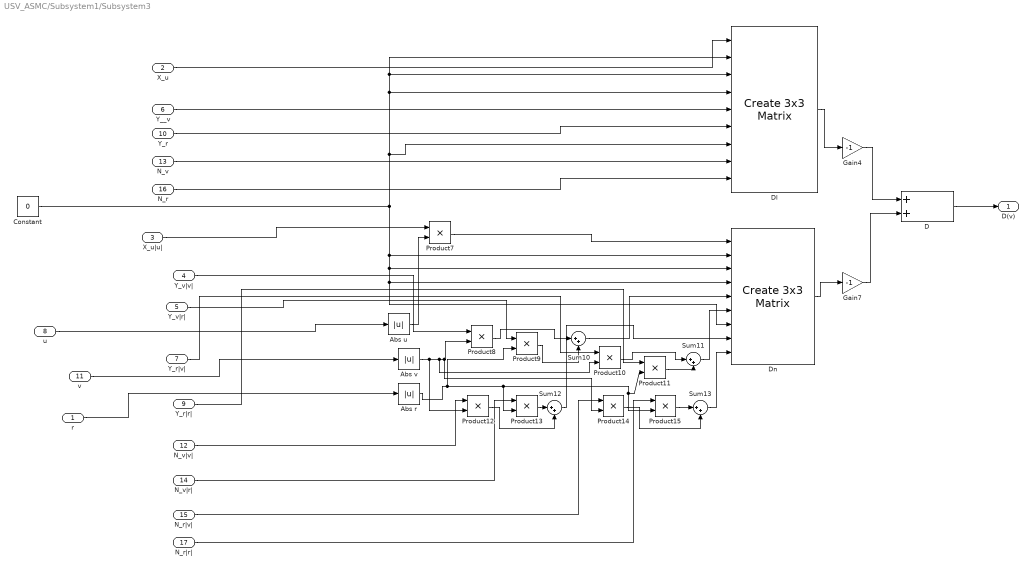
== system USV_ASMC/Subsystem1/Subsystem3 ==
  r : Inport
  X_u : Inport  Port=2
  X_u|u| : Inport  Port=3
  Y_v|v| : Inport  Port=4
  Y_v|r| : Inport  Port=5
  Y__v : Inport  Port=6
  Y_r|v| : Inport  Port=7
  u : Inport  Port=8
  Y_r|r| : Inport  Port=9
  Y_r : Inport  Port=10
  v : Inport  Port=11
  N_v|v| : Inport  Port=12
  N_v : Inport  Port=13
  N_v|r| : Inport  Port=14
  N_r|v| : Inport  Port=15
  N_r : Inport  Port=16
  N_r|r| : Inport  Port=17
  Abs r : Abs
  Abs u : Abs
  Abs v : Abs
  Constant : Constant  Value=0
  D : Sum
  Dl : sharedutil/Create 3x3 Matrix  aMode=aMode
  Dn : sharedutil/Create 3x3 Matrix  aMode=aMode
  Gain4 : Gain  Gain=-1
  Gain7 : Gain  Gain=-1
  Product{7..15} (9 alike) : Product
  Sum{10..13} (4 alike) : Sum  Inputs=|++
  D(v) : Outport  VectorParamsAs1DForOutWhenUnconnected=off
  wires:
  Constant/1 -> Dl/2, Dl/3, Dl/4, Dl/7, Dn/7, Dn/4, Dn/3, Dn/2
  Product10/1 -> Sum11/1
  Abs u/1 -> Product7/2
  Abs r/1 -> Product13/2, Product11/2, Product15/2, Product9/2
  Y_r|r|/1 -> Product11/1
  Y_v|r|/1 -> Product9/1
  Product7/1 -> Dn/1
  Sum12/1 -> Dn/8
  Abs v/1 -> Product12/2, Product10/2, Product14/2, Product8/2
  Gain7/1 -> D/2
  Y__v/1 -> Dl/5
  Product14/1 -> Sum13/2
  Gain4/1 -> D/1
  Product9/1 -> Sum10/2
  Dl/1 -> Gain4/1
  Dn/1 -> Gain7/1
  Sum10/1 -> Dn/5
  Product12/1 -> Sum12/2
  Product11/1 -> Sum11/2
  Sum13/1 -> Dn/9
  Product13/1 -> Sum12/1
  Sum11/1 -> Dn/6
  Product15/1 -> Sum13/1
  Product8/1 -> Sum10/1
  N_r/1 -> Dl/9
  r/1 -> Abs r/1
  N_v|r|/1 -> Product13/1
  X_u|u|/1 -> Product7/1
  Y_r|v|/1 -> Product10/1
  N_v|v|/1 -> Product12/1
  v/1 -> Abs v/1
  u/1 -> Abs u/1
  Y_v|v|/1 -> Product8/1
  Y_r/1 -> Dl/6
  N_r|v|/1 -> Product14/1
  N_r|r|/1 -> Product15/1
  N_v/1 -> Dl/8
  D/1 -> D(v)/1
  X_u/1 -> Dl/1

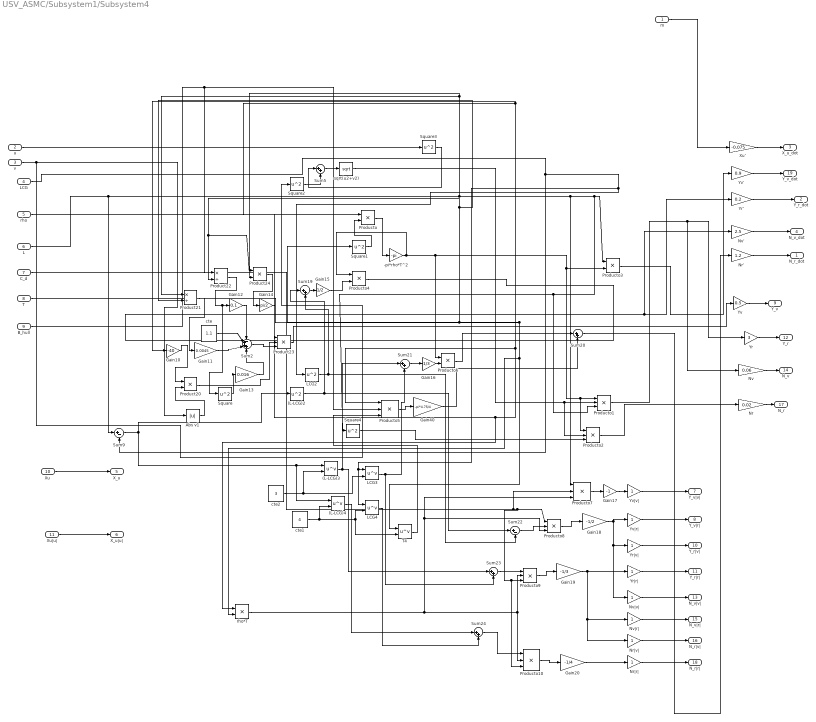
== system USV_ASMC/Subsystem1/Subsystem4 ==
  m : Inport
  u : Inport  Port=2
  v : Inport  Port=3
  LCG : Inport  Port=4
  rho : Inport  Port=5
  L : Inport  Port=6
  C_d : Inport  Port=7
  T : Inport  Port=8
  B_hull : Inport  Port=9
  Xu : Inport  Port=10
  Xu|u| : Inport  Port=11
  (L-LCG)2 : Math  Operator=square  SaturateOnIntegerOverflow=on
  (L-LCG)3 : Math  Operator=pow  SaturateOnIntegerOverflow=on
  (L-LCG)4 : Math  Operator=pow  SaturateOnIntegerOverflow=on
  -pi*rho*T^2 : Gain  Gain=-pi
  Abs v1 : Abs
  Gain10 : Gain  Gain=-40
  Gain11 : Gain  Gain=0.0045
  Gain12 : Gain  Gain=0.1
  Gain13 : Gain  Gain=0.016
  Gain14 : Gain  Gain=pi/2
  Gain15 : Gain  Gain=1/2
  Gain16 : Gain  Gain=1/3
  Gain17 : Gain  Gain=-1
  Gain18 : Gain  Gain=-1/2
  Gain19 : Gain  Gain=-1/3
  Gain20 : Gain  Gain=-1/4
  Gain40 : Gain  Gain=-pi*4.75/4
  LCG2 : Math  Operator=square  SaturateOnIntegerOverflow=on
  LCG3 : Math  Operator=pow  SaturateOnIntegerOverflow=on
  LCG4 : Math  Operator=pow  SaturateOnIntegerOverflow=on
  Nr : Gain  Gain=0.02
  Nr' : Gain  Gain=1.2
  Nr|r| : Gain
  Nr|v| : Gain
  Nv : Gain  Gain=0.06
  Nv' : Gain  Gain=2.5
  Nv|r| : Gain
  Nv|v| : Gain
  Product20 : Product
  Product21 : Product  Inputs=*/
  Product22 : Product  Inputs=*/
  Product23 : Product  Inputs=3
  Product24 : Product
  Producto{,3..4,6} (4 alike) : Product
  Producto{1..2,5,7..10} (7 alike) : Product  Inputs=3
  Square{,1..4} (5 alike) : Math  Operator=square  SaturateOnIntegerOverflow=on
  Sum{5,19..21,23..24} (6 alike) : Sum  Inputs=|++
  Sum2 : Sum  Inputs=-+++
  Sum22 : Sum  Inputs=|+-
  Sum9 : Sum  Inputs=|+-
  T4 : Math  Operator=pow  SaturateOnIntegerOverflow=on
  Xu' : Gain  Gain=-0.075
  Yr : Gain  Gain=3
  Yr' : Gain  Gain=0.2
  Yr|r| : Gain
  Yr|v| : Gain
  Yv : Gain  Gain=0.5
  Yv' : Gain  Gain=0.9
  Yv|r| : Gain
  Yv|v| : Gain
  cte : Constant  Value=1.1
  cte1 : Constant  Value=4
  cte2 : Constant  Value=3
  rho*T : Product
  sqrt(u2+v2) : Sqrt  SaturateOnIntegerOverflow=on
  N_r_dot : Outport  VectorParamsAs1DForOutWhenUnconnected=off
  Y_r_dot : Outport  Port=2  VectorParamsAs1DForOutWhenUnconnected=off
  X_u_dot : Outport  Port=3  VectorParamsAs1DForOutWhenUnconnected=off
  N_v_dot : Outport  Port=4  VectorParamsAs1DForOutWhenUnconnected=off
  X_u : Outport  Port=5  VectorParamsAs1DForOutWhenUnconnected=off
  X_u|u| : Outport  Port=6  VectorParamsAs1DForOutWhenUnconnected=off
  Y_v|v| : Outport  Port=7  VectorParamsAs1DForOutWhenUnconnected=off
  Y_v|r| : Outport  Port=8  VectorParamsAs1DForOutWhenUnconnected=off
  Y_v : Outport  Port=9  VectorParamsAs1DForOutWhenUnconnected=off
  Y_r|v| : Outport  Port=10  VectorParamsAs1DForOutWhenUnconnected=off
  Y_r|r| : Outport  Port=11  VectorParamsAs1DForOutWhenUnconnected=off
  Y_r : Outport  Port=12  VectorParamsAs1DForOutWhenUnconnected=off
  N_v|v| : Outport  Port=13  VectorParamsAs1DForOutWhenUnconnected=off
  N_v : Outport  Port=14  VectorParamsAs1DForOutWhenUnconnected=off
  N_v|r| : Outport  Port=15  VectorParamsAs1DForOutWhenUnconnected=off
  N_r|v| : Outport  Port=16  VectorParamsAs1DForOutWhenUnconnected=off
  N_r : Outport  Port=17  VectorParamsAs1DForOutWhenUnconnected=off
  N_r|r| : Outport  Port=18  VectorParamsAs1DForOutWhenUnconnected=off
  Y_v_dot : Outport  Port=19  VectorParamsAs1DForOutWhenUnconnected=off
  wires:
  C_d/1 -> Producto8/1, Producto9/3, Producto10/3, Producto7/2
  L/1 -> Producto3/1, Producto1/3, Square4/1, Producto7/1, Product24/1, Product21/1, Sum9/1
  T/1 -> T4/1, rho*T/2, Product24/2, Product22/2, Product21/2, Square1/1
  rho*T/1 -> Producto8/3, Producto7/3, Producto10/2, Producto9/2
  Gain15/1 -> Producto4/2
  Producto5/1 -> Gain40/1
  -pi*rho*T^2/1 -> Producto4/1, Producto6/1, Producto3/2, Producto2/1, Producto1/1
  Nv|r|/1 -> N_v|r|/1
  Producto/1 -> -pi*rho*T^2/1
  LCG/1 -> LCG4/1, LCG3/1, LCG2/1, Sum9/2
  LCG2/1 -> Sum22/2, Sum19/2
  Product22/1 -> Square/1, Gain12/1
  Producto1/1 -> Yr/1, Nv/1
  Nv/1 -> N_v/1
  (L-LCG)2/1 -> Sum22/1, Sum19/1
  Gain17/1 -> Yv|v|/1
  Product21/1 -> Gain11/1
  Abs v1/1 -> Product20/2
  rho/1 -> Producto5/1, Producto/1, Gain10/1, rho*T/1
  Sum5/1 -> sqrt(u2+v2)/1
  Square3/1 -> Sum5/1
  v/1 -> Square2/1, Abs v1/1
  Sum19/1 -> Gain15/1
  Producto4/1 -> Nv'/1, Yr'/1
  Gain40/1 -> Sum20/2
  T4/1 -> Producto5/3
  LCG3/1 -> Sum23/2, Sum21/2
  Producto2/1 -> Nr/1
  Square1/1 -> Producto/2
  Gain11/1 -> Sum2/3
  Producto9/1 -> Gain19/1
  Producto7/1 -> Gain17/1
  Yr'/1 -> Y_r_dot/1
  Gain18/1 -> Yv|r|/1, Nv|v|/1, Yr|v|/1
  Gain20/1 -> Nr|r|/1
  Sum23/1 -> Producto9/1
  Producto8/1 -> Gain18/1
  cte/1 -> Sum2/2
  Product23/1 -> Yv/1
  cte2/1 -> LCG3/2, (L-LCG)3/2
  cte1/1 -> T4/2, LCG4/2, (L-LCG)4/2
  Gain10/1 -> Product20/1
  Nr|v|/1 -> N_r|v|/1
  Producto3/1 -> Yv'/1
  Sum22/1 -> Producto8/2
  Gain16/1 -> Producto6/2
  Gain19/1 -> Nr|v|/1, Nv|r|/1, Yr|r|/1
  Producto6/1 -> Sum20/1
  (L-LCG)3/1 -> Sum23/1, Sum21/1
  Producto10/1 -> Gain20/1
  Sum2/1 -> Product23/3
  (L-LCG)4/1 -> Sum24/1
  Sum24/1 -> Producto10/1
  u/1 -> Square3/1
  LCG4/1 -> Sum24/2
  Sum21/1 -> Gain16/1
  Gain12/1 -> Sum2/1
  Sum20/1 -> Nr'/1
  Square2/1 -> Sum5/2
  B_hull/1 -> Producto5/2, Product22/1
  Gain13/1 -> Sum2/4
  Product20/1 -> Product23/2
  sqrt(u2+v2)/1 -> Producto2/2, Producto1/2
  Square4/1 -> Producto2/3
  Sum9/1 -> (L-LCG)4/1, (L-LCG)3/1, (L-LCG)2/1
  Product24/1 -> Gain14/1
  Nr|r|/1 -> N_r|r|/1
  Gain14/1 -> Product23/1
  Square/1 -> Gain13/1
  Nr'/1 -> N_r_dot/1
  Yr|r|/1 -> Y_r|r|/1
  Yv/1 -> Y_v/1
  Yr|v|/1 -> Y_r|v|/1
  Yv|r|/1 -> Y_v|r|/1
  Yv|v|/1 -> Y_v|v|/1
  Yr/1 -> Y_r/1
  Nr/1 -> N_r/1
  Nv|v|/1 -> N_v|v|/1
  Xu'/1 -> X_u_dot/1
  Yv'/1 -> Y_v_dot/1
  Nv'/1 -> N_v_dot/1
  m/1 -> Xu'/1
  Xu/1 -> X_u/1
  Xu|u|/1 -> X_u|u|/1

== system USV_ASMC/Subsystem1/Subsystem5 ==
  psi : Inport
  " J(n)" : sharedutil/Create 3x3 Matrix  aMode=aMode
  Constant1 : Constant
  Constant2 : Constant  Value=0
  Gain9 : Gain  Gain=-1
  Trigonometric Function : Trigonometry
  Trigonometric Function1 : Trigonometry  Operator=cos
  J(n) : Outport  VectorParamsAs1DForOutWhenUnconnected=off
  wires:
  Gain9/1 -> " J(n)"/2
  Trigonometric Function1/1 -> " J(n)"/5, " J(n)"/1
  Trigonometric Function/1 -> " J(n)"/4, Gain9/1
  Constant1/1 -> " J(n)"/9
  psi/1 -> Trigonometric Function/1, Trigonometric Function1/1
  " J(n)"/1 -> J(n)/1
  Constant2/1 -> " J(n)"/8, " J(n)"/7, " J(n)"/6, " J(n)"/3

== system USV_ASMC/Tx/(m-Yv')vr ==
  m : Inport
  Yv' : Inport  Port=2
  v : Inport  Port=3
  r : Inport  Port=4
  Product : Product  Inputs=3
  m-Yv' : Sum  Inputs=+-
  (m-Yv')vr : Outport  VectorParamsAs1DForOutWhenUnconnected=off
  wires:
  Yv'/1 -> m-Yv'/2
  v/1 -> Product/2
  m-Yv'/1 -> Product/1
  r/1 -> Product/3
  Product/1 -> (m-Yv')vr/1
  m/1 -> m-Yv'/1

== system USV_ASMC/Tx/Xdrag ==
  u : Inport
  Xu : Inport  Port=2
  Xu|u| : Inport  Port=3
  Abs : Abs
  Add : Sum
  Product : Product  Inputs=3
  Product1 : Product
  Xdrag : Outport  VectorParamsAs1DForOutWhenUnconnected=off
  wires:
  Add/1 -> Xdrag/1
  Xu|u|/1 -> Product/1
  Product/1 -> Add/1
  Xu/1 -> Product1/1
  Product1/1 -> Add/2
  Abs/1 -> Product1/2, Product/2
  u/1 -> Product/3, Abs/1

== system USV_ASMC/Tz/(-Xu'+Yv')uv ==
  Xu' : Inport
  Yv' : Inport  Port=2
  v : Inport  Port=3
  u : Inport  Port=4
  -Xu'+Yv' : Sum  Inputs=-+
  Product : Product  Inputs=3
  (-Xu'+Yv')uv : Outport  VectorParamsAs1DForOutWhenUnconnected=off
  wires:
  Yv'/1 -> -Xu'+Yv'/2
  v/1 -> Product/3
  -Xu'+Yv'/1 -> Product/1
  u/1 -> Product/2
  Product/1 -> (-Xu'+Yv')uv/1
  Xu'/1 -> -Xu'+Yv'/1

== system USV_ASMC/Tz/Nrr ==
  r : Inport
  Nr : Inport  Port=2
  Product1 : Product
  Nrr : Outport  VectorParamsAs1DForOutWhenUnconnected=off
  wires:
  Product1/1 -> Nrr/1
  Nr/1 -> Product1/1
  r/1 -> Product1/2
